simulink model "ds_cdmat2"  (Simulink 5.1)
settings: Solver=ode45  StartTime=0.0  StopTime=3  RelTol=1e-3
values from neighbouring files (symbols this model uses):
  k = [1:63]'    [DSsynf.m]
  snr = [-8:2:8]    [ds_t_m.m]
libraries: commdigbbndpm2 x4, commchan2 x2, commseqgen2 x2, dspbuff3 x2, dspsigops x1, commsink2 x1, commrandsrc2 x1, simulink x1, dspindex x1
settings Model: LastModifiedBy=Administrator  BooleanDataType=on  ProdHWDeviceType=Microprocessor

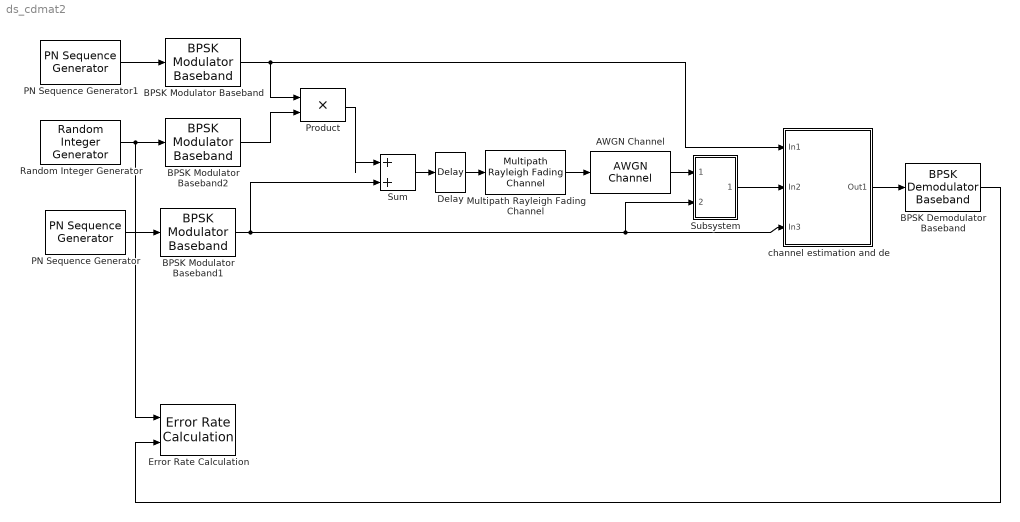
== system ds_cdmat2 ==
  AWGN Channel : commchan2/AWGN Channel  seed=67  noiseMode="Signal to noise ratio  (SNR)"  EsNodB=3  SNRdB=snr(k)  Ps=1  Tsym=1e-3/63  variance=1
  BPSK Demodulator Baseband : commdigbbndpm2/BPSK Demodulator Baseband  Ph=0  numSamp=1
  BPSK Modulator Baseband : commdigbbndpm2/BPSK Modulator Baseband  Ph=0  numSamp=1
  BPSK Modulator Baseband1 : commdigbbndpm2/BPSK Modulator Baseband  Ph=0  numSamp=1
  BPSK Modulator Baseband2 : commdigbbndpm2/BPSK Modulator Baseband  Ph=0  numSamp=1
  Delay : dspsigops/Delay  dly_unit=Samples  delay=15  ic_detail=off  dif_ic_for_ch=off  dif_ic_for_dly=off  ic=0  reset_popup=None
  Error Rate Calculation : commsink2/Error Rate Calculation  N=1  st_delay=0  cp_mode=Entire frame  subframe=[]  PMode=Workspace  WsName=ErrorVec  RsMode2=off  stop=off  numErr=100  maxBits=1e6
  Multipath Rayleigh Fading Channel : commchan2/Multipath Rayleigh Fading Channel  Fd=100  simTs=1e-3/63  delayVec=[0 6e-3/63 9e-3/63]  gainVecdB=[0 -1 -2]  normGain=off  Seed=73
  PN Sequence Generator : commseqgen2/PN Sequence Generator  poly=[1 1 0 0 1 1 1]  ini_sta="[0 0 0 0  0 1]"  shift=0  Ts=1e-3/63  frameBased=on  sampPerFrame=63  reset=off
  PN Sequence Generator1 : commseqgen2/PN Sequence Generator  poly=[1 0 0 0 0 1 1]  ini_sta=[0 0 0 0 0 1]  shift=0  Ts=1e-3/63  frameBased=on  sampPerFrame=63  reset=off
  Product : Product  SaturateOnIntegerOverflow=on
  Random Integer Generator : commrandsrc2/Random Integer Generator  mul=2  seed=37  Ts=1e-3  frameBased=on  sampPerFrame=1  orient=off
  Subsystem : Subsystem
  Sum : Sum  Inputs=|++  SaturateOnIntegerOverflow=on
  channel estimation and de : Subsystem
  wires:
  Random Integer Generator/1 -> BPSK Modulator Baseband2/1, Error Rate Calculation/1
  PN Sequence Generator1/1 -> BPSK Modulator Baseband/1
  PN Sequence Generator/1 -> BPSK Modulator Baseband1/1
  BPSK Modulator Baseband/1 -> Product/1, channel estimation and de/1(In1)
  BPSK Modulator Baseband2/1 -> Product/2
  BPSK Modulator Baseband1/1 -> channel estimation and de/3(In3), Subsystem/2(In2), Sum/2
  Multipath Rayleigh Fading Channel/1 -> AWGN Channel/1
  BPSK Demodulator Baseband/1 -> Error Rate Calculation/2
  AWGN Channel/1 -> Subsystem/1(In1)
  channel estimation and de/1(Out1) -> BPSK Demodulator Baseband/1
  Subsystem/1(Out1) -> channel estimation and de/2(In2)
  Delay/1 -> Multipath Rayleigh Fading Channel/1
  Sum/1 -> Delay/1
  Product/1 -> Sum/1

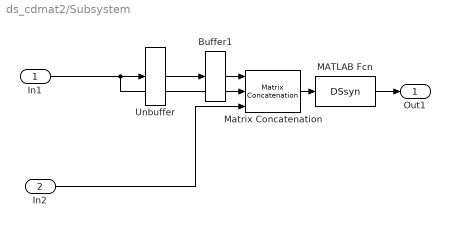
== system ds_cdmat2/Subsystem ==
  In1 : Inport
  In2 : Inport  Port=2
  Buffer1 : dspbuff3/Buffer  N=63  V=0  ic=0
  MATLAB Fcn : MATLABFcn  MATLABFcn=DSsyn  Output1D=off
  Matrix Concatenation : simulink/Math Operations/Matrix Concatenation  numInports=3  catMethod=Vertical
  Unbuffer : dspbuff3/Unbuffer  ic=0
  Out1 : Outport
  wires:
  Buffer1/1 -> Matrix Concatenation/1
  Matrix Concatenation/1 -> MATLAB Fcn/1
  In2/1 -> Matrix Concatenation/3
  In1/1 -> Unbuffer/1, Matrix Concatenation/2
  MATLAB Fcn/1 -> Out1/1
  Unbuffer/1 -> Buffer1/1

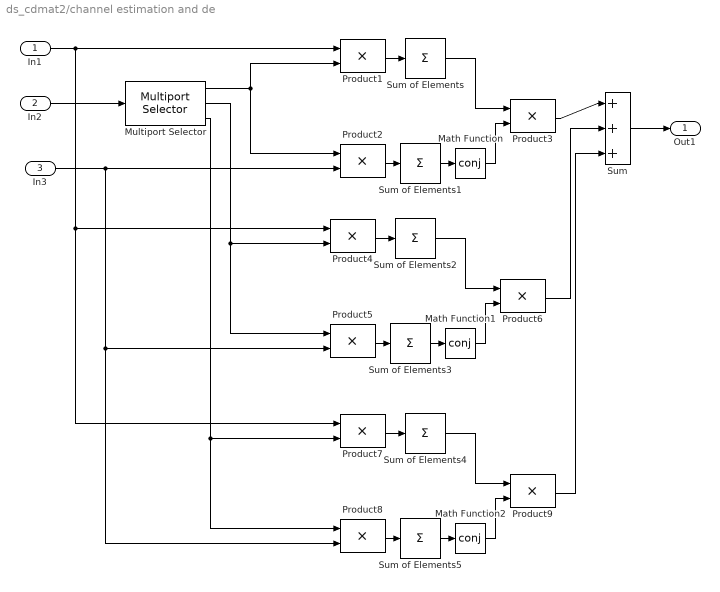
== system ds_cdmat2/channel estimation and de ==
  In1 : Inport
  In2 : Inport  Port=2
  In3 : Inport  Port=3
  Math Function : Math  Operator=conj
  Math Function1 : Math  Operator=conj
  Math Function2 : Math  Operator=conj
  Multiport Selector : dspindex/Multiport Selector  rowsOrCols=Rows  idxCellArray={[1:63], [64:126],[127:189] }  idxErrMode=Clip Index
  Product{1..9} (9 alike) : Product  SaturateOnIntegerOverflow=on
  Sum : Sum  Inputs=|+++  ShowAdditionalParam=on  SaturateOnIntegerOverflow=on
  Sum of Elements{,1..5} (6 alike) : Sum  Inputs=+  ShowAdditionalParam=on  OutScaling=2^-10
  Out1 : Outport
  wires:
  Sum of Elements1/1 -> Math Function/1
  Product2/1 -> Sum of Elements1/1
  Sum of Elements/1 -> Product3/1
  Product1/1 -> Sum of Elements/1
  In1/1 -> Product1/1, Product4/1, Product7/1
  In3/1 -> Product2/2, Product5/2, Product8/2
  Math Function/1 -> Product3/2
  In2/1 -> Multiport Selector/1
  Multiport Selector/1 -> Product1/2, Product2/1
  Sum of Elements3/1 -> Math Function1/1
  Product5/1 -> Sum of Elements3/1
  Sum of Elements2/1 -> Product6/1
  Product4/1 -> Sum of Elements2/1
  Math Function1/1 -> Product6/2
  Sum of Elements5/1 -> Math Function2/1
  Product8/1 -> Sum of Elements5/1
  Sum of Elements4/1 -> Product9/1
  Product7/1 -> Sum of Elements4/1
  Math Function2/1 -> Product9/2
  Multiport Selector/2 -> Product4/2, Product5/1
  Multiport Selector/3 -> Product7/2, Product8/1
  Sum/1 -> Out1/1
  Product3/1 -> Sum/1
  Product9/1 -> Sum/3
  Product6/1 -> Sum/2
